simulink model "chache_jizuobiao"  (R2022a)
settings: Solver=VariableStepAuto  StartTime=0.0  StopTime=100  RelTol=1e-3
settings Model: Creator=18222  LastModifiedBy=18222

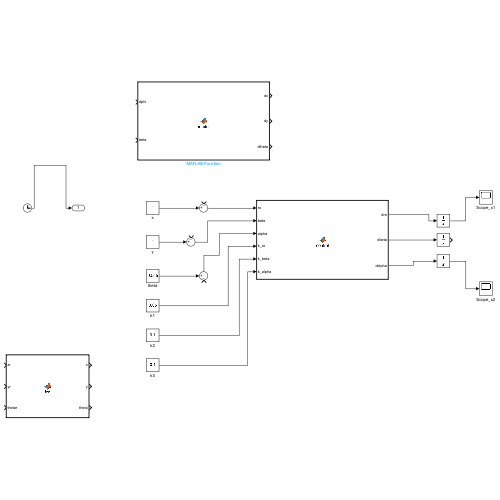
[thumbnail: Simulink's stored preview of the top-level diagram]
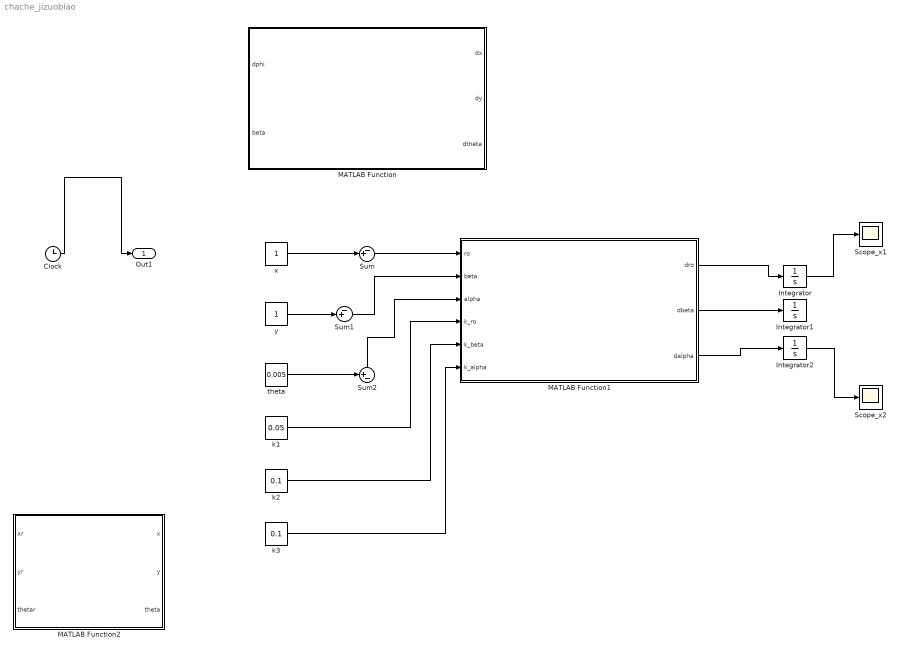
== system chache_jizuobiao ==
  Clock : Clock
  Integrator : Integrator
  Integrator1 : Integrator
  Integrator2 : Integrator
  MATLAB Function : MATLAB Function  TreatAsAtomicUnit=on
  MATLAB Function1 : MATLAB Function  TreatAsAtomicUnit=on
  MATLAB Function2 : MATLAB Function  TreatAsAtomicUnit=on
  Scope_x1 : Scope
  Scope_x2 : Scope
  Sum : Sum  Inputs=-+|
  Sum1 : Sum  Inputs=-+|
  Sum2 : Sum  Inputs=+-|
  k1 : Constant  Value=0.05
  k2 : Constant  Value=0.1
  k3 : Constant  Value=0.1
  theta : Constant  Value=0.005
  x : Constant
  y : Constant
  Out1 : Outport
  wires:
  x/1 -> Sum/2
  Sum/1 -> MATLAB Function1/1(ro)
  Clock/1 -> Out1/1
  y/1 -> Sum1/2
  theta/1 -> Sum2/1
  Sum1/1 -> MATLAB Function1/2(beta)
  Sum2/1 -> MATLAB Function1/3(alpha)
  k1/1 -> MATLAB Function1/4(k_ro)
  k2/1 -> MATLAB Function1/5(k_beta)
  MATLAB Function1/1(dro) -> Integrator/1
  MATLAB Function1/2(dbeta) -> Integrator1/1
  Integrator2/1 -> Scope_x2/1
  Integrator/1 -> Scope_x1/1
  MATLAB Function1/3(dalpha) -> Integrator2/1
  k3/1 -> MATLAB Function1/6(k_alpha)

== matlab function chache_jizuobiao/MATLAB Function1 ==
  data: ro input; dro output; beta input; dbeta output; alpha input; k_ro input; k_beta input; k_alpha input; dalpha output
function [dro, dbeta, dalpha] = control(ro, beta, alpha, k_ro, k_beta, k_alpha)
dro = -k_ro*ro*cos(alpha);
dbeta = -k_ro * sin(alpha);
dalpha = k_ro * sin(alpha) - k_alpha*alpha - k_beta*beta;

== matlab function chache_jizuobiao/MATLAB Function ==
  data: dphi input; dx output; beta input; dy output; dtheta output
function [dx, dy, dtheta] = model(dphi, beta)
R = 1;
L2 = 2;
dx = R*dphi*sin(beta);
dy = 0;
dtheta = -R*dphi*cos(beta)/L2;

== matlab function chache_jizuobiao/MATLAB Function2 ==
  data: x output; xr input; y output; yr input; thetar input; theta output
function [x, y, theta] = fcn(xr, yr, thetar)
theta = thetar;
R=[cos(theta) sin(theta) 0;
    -sin(theta) cos(theta) 0;
    0 0 1];

result = inv(R)*[xr;yr;thetar];
x = result(1);
y = result(2);
